simulink model "ClosedLoop_LQR"  (R2024a)
settings: Solver=VariableStepAuto  StartTime=0.0  StopTime=10.0  RelTol=1e-3
values from neighbouring files (symbols this model uses):
  A = a    [rscale.m]
  B = b    [rscale.m]
  C = c    [rscale.m]
undefined symbols (not defined in the file or in its folder): K_lqr, N_bar_lqr
settings Model: Creator=mahariansyah  LastModifiedBy=mahariansyah

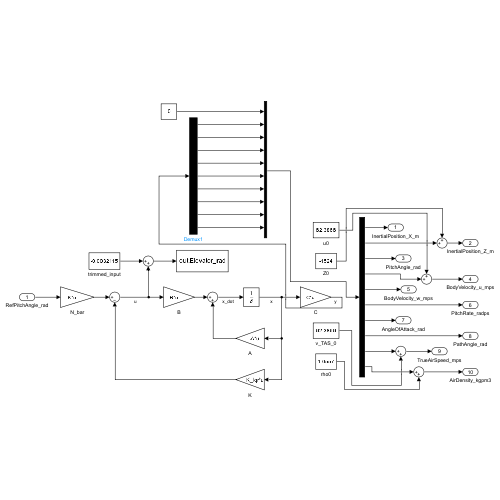
[thumbnail: Simulink's stored preview of the top-level diagram]
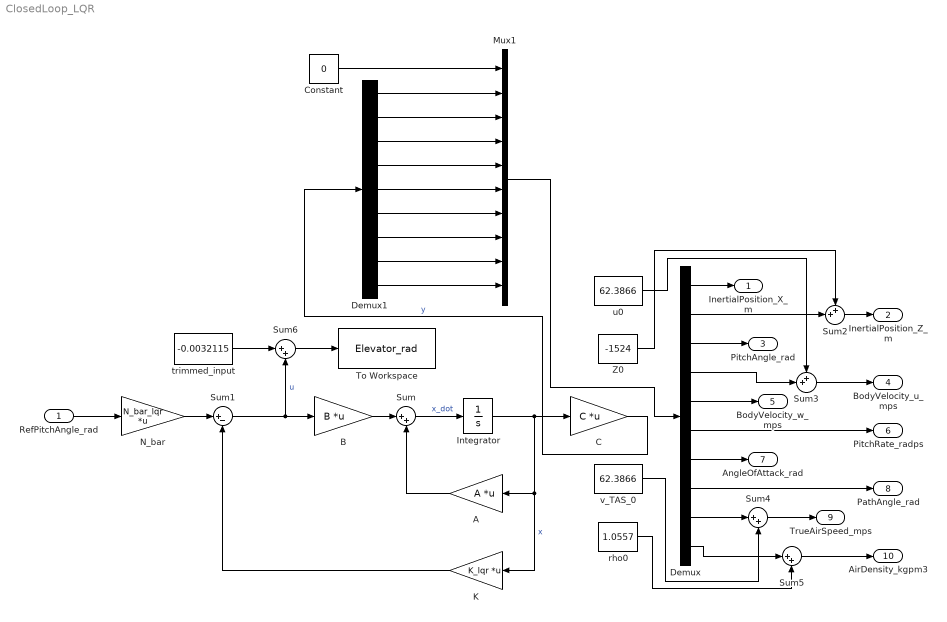
== system ClosedLoop_LQR ==
  RefPitchAngle_rad : Inport
  A : Gain  Gain=A  Multiplication=Matrix(K*u)
  B : Gain  Gain=B  Multiplication=Matrix(K*u)
  C : Gain  Gain=C  Multiplication=Matrix(K*u)
  Constant : Constant  Value=0
  Demux : Demux  Outputs=10
  Demux1 : Demux  Outputs=9
  Integrator : Integrator
  K : Gain  Gain=K_lqr  Multiplication=Matrix(K*u)
  Mux1 : Mux  Inputs=10
  N_bar : Gain  Gain=N_bar_lqr  Multiplication=Matrix(K*u)
  Sum{,4..6} (4 alike) : Sum  Inputs=|++
  Sum1 : Sum  Inputs=|+-
  Sum2 : Sum  Inputs=++|
  Sum3 : Sum  Inputs=++|
  To Workspace : ToWorkspace  VariableName=Elevator_rad  SaveFormat=Timeseries  SampleTime=-1
  Z0 : Constant  Value=-1524
  rho0 : Constant  Value=1.0557
  trimmed_input : Constant  Value=-0.0032115
  u0 : Constant  Value=62.3866
  v_TAS_0 : Constant  Value=62.3866
  InertialPosition_X_m : Outport
  InertialPosition_Z_m : Outport  Port=2
  PitchAngle_rad : Outport  Port=3
  BodyVelocity_u_mps : Outport  Port=4
  BodyVelocity_w_mps : Outport  Port=5
  PitchRate_radps : Outport  Port=6
  AngleOfAttack_rad : Outport  Port=7
  PathAngle_rad : Outport  Port=8
  TrueAirSpeed_mps : Outport  Port=9
  AirDensity_kgpm3 : Outport  Port=10
  wires:
  Integrator/1 -> K/1, A/1, C/1  "x"
  Sum/1 -> Integrator/1  "x_dot"
  A/1 -> Sum/2
  B/1 -> Sum/1
  Sum1/1 -> B/1, Sum6/2  "u"
  RefPitchAngle_rad/1 -> N_bar/1
  Demux/1 -> InertialPosition_X_m/1
  Demux/3 -> PitchAngle_rad/1
  Demux/5 -> BodyVelocity_w_mps/1
  Demux/6 -> PitchRate_radps/1
  Demux/7 -> AngleOfAttack_rad/1
  Demux/8 -> PathAngle_rad/1
  Sum2/1 -> InertialPosition_Z_m/1
  Demux/2 -> Sum2/2
  Z0/1 -> Sum2/1
  Demux/4 -> Sum3/2
  Sum3/1 -> BodyVelocity_u_mps/1
  u0/1 -> Sum3/1
  Sum4/1 -> TrueAirSpeed_mps/1
  Demux/9 -> Sum4/1
  v_TAS_0/1 -> Sum4/2
  Sum5/1 -> AirDensity_kgpm3/1
  Demux/10 -> Sum5/1
  rho0/1 -> Sum5/2
  trimmed_input/1 -> Sum6/1
  Sum6/1 -> To Workspace/1
  N_bar/1 -> Sum1/1
  K/1 -> Sum1/2
  Mux1/1 -> Demux/1
  Demux1/9 -> Mux1/10
  Demux1/8 -> Mux1/9
  Demux1/7 -> Mux1/8
  Demux1/6 -> Mux1/7
  Demux1/5 -> Mux1/6
  Demux1/4 -> Mux1/5
  Demux1/3 -> Mux1/4
  Demux1/2 -> Mux1/3
  Demux1/1 -> Mux1/2
  Constant/1 -> Mux1/1
  C/1 -> Demux1/1  "y"
